simulink model "pibit_completo_2025_sem_obs_2025_2"  (R2025a)
settings: Solver=VariableStepAuto  StartTime=0.0  StopTime=10.0  RelTol=1e-3
values from neighbouring files (symbols this model uses):
  bp = 5    [parametros_suspensao_completo_pibit.m]    (also in parametros_suspensao_completo_pibit_final.m)
  bs = 10    [parametros_suspensao_completo_pibit.m]    (also in parametros_suspensao_completo_pibit_final.m)
  g = 9.81    [parametros_suspensao_completo_pibit.m]    (also in parametros_suspensao_completo_pibit_final.m)
  I = 5.6e-4    (= 0.00056)    [parametros_suspensao_completo_pibit.m]    (also in parametros_suspensao_completo_pibit_final.m)
  I_carroceria = (1/12) * m_carroceria * (L^2 + H^2)    (= 0.0082936384875)    [parametros_suspensao_completo_pibit_final.m]
  kp = 1000    [parametros_suspensao_completo_pibit.m]    (also in parametros_suspensao_completo_pibit_final.m)
  ks = 200    [parametros_suspensao_completo_pibit.m]    (also in parametros_suspensao_completo_pibit_final.m)
  M = [ ... (first row only)    [aprimorado_matlab_function_matriz_transformacao.m]    (also in bloco_matriz_tranformacao_pibit_final.m; bloco_matriz_tranformacao_pibit_semifinal.m; bloco_transposta_matriz_transformacao.m; matlab_function_matriz_transformacao.m)
  m_carroceria = 0.598725    [parametros_suspensao_completo_pibit_final.m]
  M_transposta = M'    [bloco_transposta_matriz_transformacao.m]    (also in parametros_suspensao_completo_pibit_final.m = [1  0  1  0  1)
  massa_nao_suspensa = 200/1000    (= 0.2)    [parametros_suspensao_completo_pibit.m]    (also in parametros_suspensao_completo_pibit_final.m)
  Vv = 5    [parametros_suspensao_completo_pibit_final.m]
  z0_carroceria = 0.12    [parametros_suspensao_completo_pibit_final.m]
  z0_roda = 0.04    [parametros_suspensao_completo_pibit_final.m]

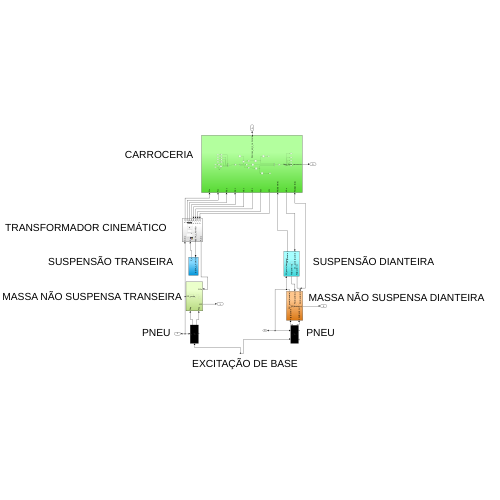
[thumbnail: Simulink's stored preview of the top-level diagram]
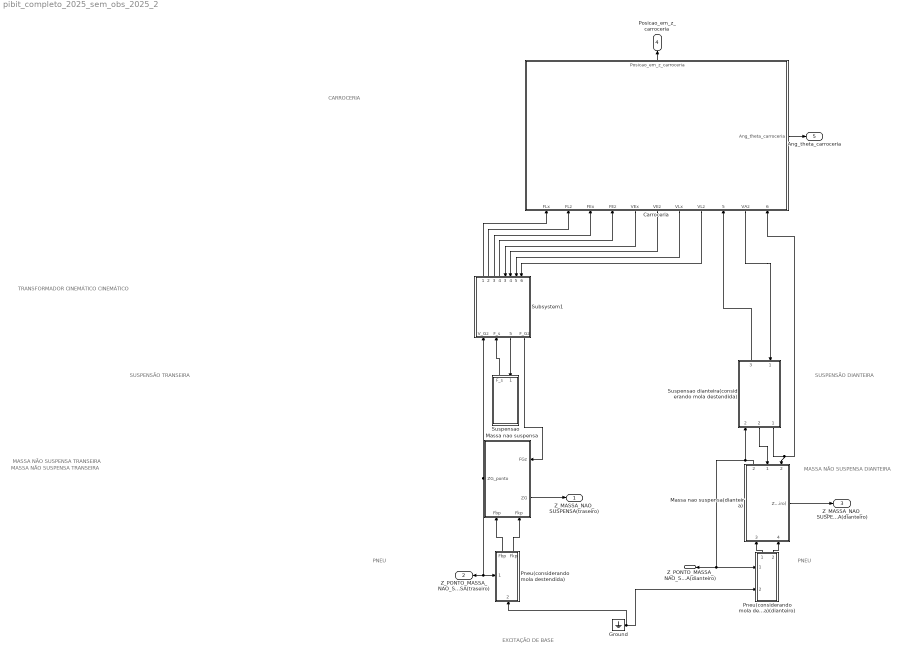
== system pibit_completo_2025_sem_obs_2025_2 ==
  note: MASSA NÃO SUSPENSA TRANSEIRA
  note: EXCITAÇÃO DE BASE
  note: SUSPENSÃO TRANSEIRA
  note: MASSA NÃO SUSPENSA DIANTEIRA
  note: SUSPENSÃO DIANTEIRA
  note: MASSA NÃO SUSPENSA TRANSEIRA
  note: CARROCERIA
  note: TRANSFORMADOR CINEMÁTICO
      |
      | CINEMÁTICO
  note: PNEU
  note: PNEU
  Carroceria : Subsystem
      settings: PortSchema="{\"entries\":[{\"content\":{\"sides\":[{\"content\":{},\"type\":\"ConnectorPlacement.EquallySpacedRectSide\",\"uuid\":\"bbb56681-fa3a-494c-b09e-961173c7fba7\"},{\"content\":{\"connectorIds\":[\"Out1\"],\"side\":\"RIGHT\"},\"type\":\"ConnectorPlacement.EquallySpacedRectSide\",\"uuid\":\"b39b7f7c-1399-4660-80c4-7db9c0d91b8e\"},{\"content\":{\"connectorIds\":[\"Out7\"],\"side\":\"TOP\"},\"type\":\"ConnectorPlacement.EquallySpacedRectSide\",\"uuid\":\"6aac35c2-b40a-442b-b0dd-a1f968c28842\"},{\"content\":{\"connectorIds\":[\"In1\",\"In2\",\"In3\",\"In4\",\"Out2\",\"Out3\",\"Out4\",\"Out5\",\"In5\",\"Out6\",\"In6\"],\"side\":\"BOTTOM\"},\"type\":\"ConnectorPlacement.EquallySpacedRectSide\",\"uuid\":\"4245813e-a678-4af8-87f3-459b1c319aee\"}]},\"type\":\"ConnectorPlacement.EquallySpacedConnector\",\"uuid\":\"f483dfe5-875a-4915-bcaf-a6efbf263f8a\"}],\"packageUris\":[\"http://schema.mathworks.com/mf0/Connector/R2020b\"],\"version\":\"1.0\"}"
  Ground : Ground
  Massa nao suspensa : Subsystem
      settings: PortSchema="{\"entries\":[{\"content\":{\"sides\":[{\"content\":{\"connectorIds\":[\"Out2\"]},\"type\":\"ConnectorPlacement.EquallySpacedRectSide\",\"uuid\":\"89344802-da43-4975-9b71-8316dc3fb6e7\"},{\"content\":{\"connectorIds\":[\"In3\",\"Out1\"],\"side\":\"RIGHT\"},\"type\":\"ConnectorPlacement.EquallySpacedRectSide\",\"uuid\":\"44d29e65-683b-44cb-8a4b-cd86ab3b5135\"},{\"content\":{\"side\":\"TOP\"},\"type\":\"ConnectorPlacement.EquallySpacedRectSide\",\"uuid\":\"980e030f-54fe-4b18-9c23-6eb2fde540e6\"},{\"content\":{\"connectorIds\":[\"In1\",\"In2\"],\"side\":\"BOTTOM\"},\"type\":\"ConnectorPlacement.EquallySpacedRectSide\",\"uuid\":\"baf76e64-0ac7-4a13-9c9f-461733e0ed7e\"}]},\"type\":\"ConnectorPlacement.EquallySpacedConnector\",\"uuid\":\"754d74c1-f226-49ce-a628-45964590b37b\"}],\"packageUris\":[\"http://schema.mathworks.com/mf0/Connector/R2020b\"],\"version\":\"1.0\"}"
  Massa nao suspensa(dianteira) : Subsystem
      settings: PortSchema="{\"entries\":[{\"content\":{\"sides\":[{\"content\":{},\"type\":\"ConnectorPlacement.EquallySpacedRectSide\",\"uuid\":\"c3cf290d-eebe-430e-95e8-be70dab148a6\"},{\"content\":{\"connectorIds\":[\"Out1\"],\"side\":\"RIGHT\"},\"type\":\"ConnectorPlacement.EquallySpacedRectSide\",\"uuid\":\"ff14580b-ed99-4b60-a1b6-b7a8b25b7868\"},{\"content\":{\"connectorIds\":[\"Out2\",\"In1\",\"In2\"],\"side\":\"TOP\"},\"type\":\"ConnectorPlacement.EquallySpacedRectSide\",\"uuid\":\"eb642ce5-fa56-48cf-87cc-3fd9675ce156\"},{\"content\":{\"connectorIds\":[\"In3\",\"In4\"],\"side\":\"BOTTOM\"},\"type\":\"ConnectorPlacement.EquallySpacedRectSide\",\"uuid\":\"0b9c6cb4-9fe7-4c64-813d-ec4cf3dc3e2a\"}]},\"type\":\"ConnectorPlacement.EquallySpacedConnector\",\"uuid\":\"a6d34252-cdb4-4e0a-800a-fcf48d8dc927\"}],\"packageUris\":[\"http://schema.mathworks.com/mf0/Connector/R2020b\"],\"version\":\"1.0\"}"
  Pneu(considerando mola destendida) : Subsystem
      settings: PortSchema="{\"entries\":[{\"content\":{\"sides\":[{\"content\":{\"connectorIds\":[\"In1\"]},\"type\":\"ConnectorPlacement.EquallySpacedRectSide\",\"uuid\":\"c5d69704-cabb-4fdd-98c1-bf4ac49d8bff\"},{\"content\":{\"side\":\"RIGHT\"},\"type\":\"ConnectorPlacement.EquallySpacedRectSide\",\"uuid\":\"557f2c7d-9be1-4292-a002-7cfc4acdfa17\"},{\"content\":{\"connectorIds\":[\"Out1\",\"Out2\"],\"side\":\"TOP\"},\"type\":\"ConnectorPlacement.EquallySpacedRectSide\",\"uuid\":\"4d76a2f1-24c8-44da-a892-d1fe66b59528\"},{\"content\":{\"connectorIds\":[\"In2\"],\"side\":\"BOTTOM\"},\"type\":\"ConnectorPlacement.EquallySpacedRectSide\",\"uuid\":\"89b6f56a-af2b-419d-a0b0-9e96ef479f92\"}]},\"type\":\"ConnectorPlacement.EquallySpacedConnector\",\"uuid\":\"f14e1ba1-d9bd-4a41-a66d-11d76b469bcb\"}],\"packageUris\":[\"http://schema.mathworks.com/mf0/Connector/R2020b\"],\"version\":\"1.0\"}"
  Pneu(considerando mola destendida)(dianteiro) : Subsystem
      settings: PortSchema="{\"entries\":[{\"content\":{\"sides\":[{\"content\":{\"connectorIds\":[\"In1\",\"In2\"]},\"type\":\"ConnectorPlacement.EquallySpacedRectSide\",\"uuid\":\"c5d69704-cabb-4fdd-98c1-bf4ac49d8bff\"},{\"content\":{\"side\":\"RIGHT\"},\"type\":\"ConnectorPlacement.EquallySpacedRectSide\",\"uuid\":\"557f2c7d-9be1-4292-a002-7cfc4acdfa17\"},{\"content\":{\"connectorIds\":[\"Out1\",\"Out2\"],\"side\":\"TOP\"},\"type\":\"ConnectorPlacement.EquallySpacedRectSide\",\"uuid\":\"4d76a2f1-24c8-44da-a892-d1fe66b59528\"}]},\"type\":\"ConnectorPlacement.EquallySpacedConnector\",\"uuid\":\"f14e1ba1-d9bd-4a41-a66d-11d76b469bcb\"}],\"packageUris\":[\"http://schema.mathworks.com/mf0/Connector/R2020b\"],\"version\":\"1.0\"}"
  Subsystem1 : Subsystem
      settings: PortSchema="{\"entries\":[{\"content\":{\"sides\":[{\"content\":{\"connectorIds\":[\"In1\",\"In2\",\"Out5\",\"Out6\"]},\"type\":\"ConnectorPlacement.EquallySpacedRectSide\",\"uuid\":\"bebb3b97-f51a-4e56-a2ac-0bf355c169a6\"},{\"content\":{\"connectorIds\":[\"Out1\",\"Out2\",\"Out3\",\"Out4\",\"In3\",\"In4\",\"In5\",\"In6\"],\"side\":\"RIGHT\"},\"type\":\"ConnectorPlacement.EquallySpacedRectSide\",\"uuid\":\"70a45981-1049-4317-936c-533ae84876c2\"},{\"content\":{\"side\":\"TOP\"},\"type\":\"ConnectorPlacement.EquallySpacedRectSide\",\"uuid\":\"f9228920-a333-4bb0-97b2-e9b2d0e5e8fb\"}]},\"type\":\"ConnectorPlacement.EquallySpacedConnector\",\"uuid\":\"080e89e8-39a4-4dac-ac05-f09c1a8f52a2\"}],\"packageUris\":[\"http://schema.mathworks.com/mf0/Connector/R2020b\"],\"version\":\"1.0\"}"
  Suspensao : Subsystem
      settings: PortSchema="{\"entries\":[{\"content\":{\"sides\":[{\"content\":{},\"type\":\"ConnectorPlacement.EquallySpacedRectSide\",\"uuid\":\"4f1921ee-033d-46ee-8e73-30eca5c2181d\"},{\"content\":{\"side\":\"RIGHT\"},\"type\":\"ConnectorPlacement.EquallySpacedRectSide\",\"uuid\":\"dda2b99d-9329-4e8f-bdf2-d73cce971ac2\"},{\"content\":{\"connectorIds\":[\"In1\",\"Out1\"],\"side\":\"TOP\"},\"type\":\"ConnectorPlacement.EquallySpacedRectSide\",\"uuid\":\"e9d42515-3d20-42dd-b281-3c9bfd9b1cfa\"},{\"content\":{\"side\":\"BOTTOM\"},\"type\":\"ConnectorPlacement.EquallySpacedRectSide\",\"uuid\":\"bd1a0df3-c979-436b-84b6-72c0af110375\"}]},\"type\":\"ConnectorPlacement.EquallySpacedConnector\",\"uuid\":\"cbab4240-af80-4068-bc0e-573c06bf1f73\"}],\"packageUris\":[\"http://schema.mathworks.com/mf0/Connector/R2020b\"],\"version\":\"1.0\"}"
  Suspensao dianteira(considerando mola destendida) : Subsystem
      settings: PortSchema="{\"entries\":[{\"content\":{\"sides\":[{\"content\":{\"connectorIds\":[\"In1\",\"Out3\"]},\"type\":\"ConnectorPlacement.EquallySpacedRectSide\",\"uuid\":\"d327c13d-9315-480e-be5c-199a2935ffa2\"},{\"content\":{\"connectorIds\":[\"Out1\",\"Out2\",\"In2\"],\"side\":\"RIGHT\"},\"type\":\"ConnectorPlacement.EquallySpacedRectSide\",\"uuid\":\"b456819d-8f70-476a-8897-c81e34c4473c\"},{\"content\":{\"side\":\"TOP\"},\"type\":\"ConnectorPlacement.EquallySpacedRectSide\",\"uuid\":\"b01201ff-aebb-430e-af55-356b9f96849b\"}]},\"type\":\"ConnectorPlacement.EquallySpacedConnector\",\"uuid\":\"690aae98-0b40-4873-810d-deff39bc59c7\"}],\"packageUris\":[\"http://schema.mathworks.com/mf0/Connector/R2020b\"],\"version\":\"1.0\"}"
  Z_MASSA_NAO_SUSPENSA(traseiro) : Outport
  Z_PONTO_MASSA_NAO_SUSPENSA(traseiro) : Outport  Port=2
  Z_MASSA_NAO_SUSPENSA(dianteiro) : Outport  Port=3
  Posicao_em_z_carroceria : Outport  Port=4
  Ang_theta_carroceria : Outport  Port=5
  Z_PONTO_MASSA_NAO_SUSPENSA(dianteiro) : Outport  Port=6
  wires:
  Subsystem1/1(F_Lx) -> Carroceria/1(FLx)
  Massa nao suspensa/1(ZG) -> Z_MASSA_NAO_SUSPENSA(traseiro)/1
  Pneu(considerando mola destendida)(dianteiro)/2(Fbp(dianteiro)) -> Massa nao suspensa(dianteira)/4(Fbp(dianteiro))
  Massa nao suspensa/2(ZG_ponto) -> Z_PONTO_MASSA_NAO_SUSPENSA(traseiro)/1, Pneu(considerando mola destendida)/1(ZG_ponto), Subsystem1/1(V_Gz)
  Suspensao dianteira(considerando mola destendida)/2(Fk(dianteiro)1) -> Massa nao suspensa(dianteira)/1(Fb(dianteiro)1)
  Suspensao/1(F_s) -> Subsystem1/2(F_s)
  Massa nao suspensa(dianteira)/2(ZG_ponto(dianteiro)) -> Suspensao dianteira(considerando mola destendida)/2(ZG_ponto(dianteiro)), Z_PONTO_MASSA_NAO_SUSPENSA(dianteiro)/1, Pneu(considerando mola destendida)(dianteiro)/1(ZG_ponto(dianteiro))
  Suspensao dianteira(considerando mola destendida)/3(Fb(dianteiro)) -> Carroceria/5(Fb(dianteiro))
  Subsystem1/6(F_Gz) -> Massa nao suspensa/3(FGz)
  Subsystem1/4(F_Ez) -> Carroceria/4(FEz)
  Subsystem1/3(F_Ex) -> Carroceria/3(FEx)
  Carroceria/1(Ang_theta_carroceria) -> Ang_theta_carroceria/1
  Carroceria/6(VAz) -> Suspensao dianteira(considerando mola destendida)/1(ZA_ponto(dianteiro))
  Carroceria/7(Posicao_em_z_carroceria) -> Posicao_em_z_carroceria/1
  Carroceria/2(VEx) -> Subsystem1/3(V_Ex)
  Pneu(considerando mola destendida)(dianteiro)/1(Fkp(dianteiro)) -> Massa nao suspensa(dianteira)/3(Fkp(dianteiro))
  Carroceria/5(VLz) -> Subsystem1/6(V_Lz)
  Carroceria/4(VLx) -> Subsystem1/5(V_Lx)
  Suspensao dianteira(considerando mola destendida)/1(Fk(dianteiro)) -> Massa nao suspensa(dianteira)/2(Fk(dianteiro)2), Carroceria/6(Fk(dianteiro))
  Carroceria/3(VEz) -> Subsystem1/4(V_Ez)
  Subsystem1/5(BETA_1_PONTO) -> Suspensao/1(BETA_1_PONTO)
  Massa nao suspensa(dianteira)/1(ZG(dianteiro)) -> Z_MASSA_NAO_SUSPENSA(dianteiro)/1
  Pneu(considerando mola destendida)/2(Fkp) -> Massa nao suspensa/2(Fkp)
  Subsystem1/2(F_Lz) -> Carroceria/2(FLz)
  Pneu(considerando mola destendida)/1(Fbp) -> Massa nao suspensa/1(Fbp)
  Ground/1 -> Pneu(considerando mola destendida)/2(Z1_ponto), Pneu(considerando mola destendida)(dianteiro)/2(Z1_ponto(dianteiro))

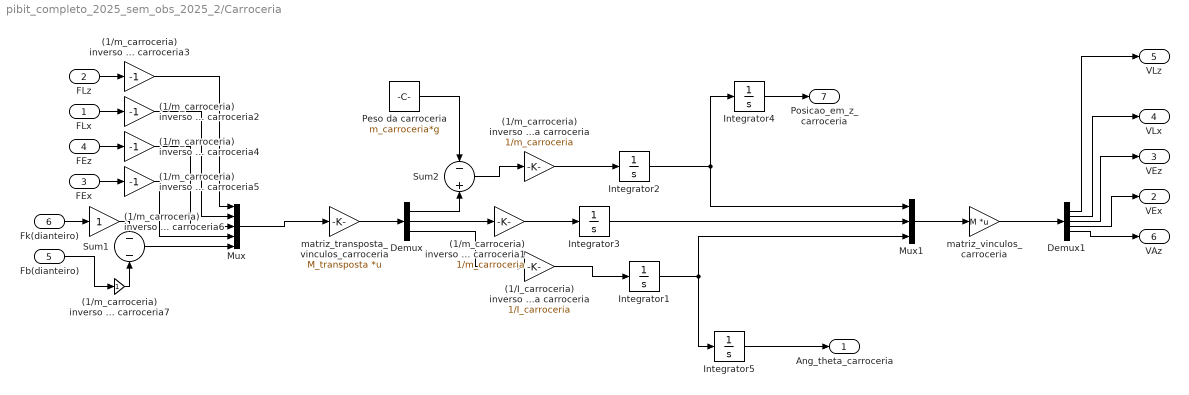
== system pibit_completo_2025_sem_obs_2025_2/Carroceria ==
  FLx : Inport
  FLz : Inport  Port=2
  FEx : Inport  Port=3
  FEz : Inport  Port=4
  Fb(dianteiro) : Inport  Port=5
  Fk(dianteiro) : Inport  Port=6
  (1/I_carroceria) inverso do momento de inercia da carroceria : Gain  Gain=1/I_carroceria
  (1/m_carroceria) inverso da massa da carroceria : Gain  Gain=1/m_carroceria
  (1/m_carroceria) inverso da massa da carroceria1 : Gain  Gain=1/m_carroceria
  (1/m_carroceria) inverso da massa da carroceria{2..5} (4 alike) : Gain  Gain=-1
  (1/m_carroceria) inverso da massa da carroceria6 : Gain
  (1/m_carroceria) inverso da massa da carroceria7 : Gain
  Demux : Demux  Outputs=3
  Demux1 : Demux  Outputs=5
  Integrator1 : Integrator
  Integrator2 : Integrator
  Integrator3 : Integrator  InitialCondition=Vv
  Integrator4 : Integrator  InitialCondition=z0_carroceria
  Integrator5 : Integrator
  Mux : Mux  Inputs=5
  Mux1 : Mux  Inputs=3
  Peso da carroceria : Constant  Value=m_carroceria*g
  Sum1 : Sum  Inputs=--
  Sum2 : Sum  Inputs=-+
  matriz_transposta_vinculos_carroceria : Gain  Gain=M_transposta  Multiplication=Matrix(K*u) (u vector)
  matriz_vinculos_carroceria : Gain  Gain=M  Multiplication=Matrix(K*u) (u vector)
  Ang_theta_carroceria : Outport
  VEx : Outport  Port=2
  VEz : Outport  Port=3
  VLx : Outport  Port=4
  VLz : Outport  Port=5
  VAz : Outport  Port=6
  Posicao_em_z_carroceria : Outport  Port=7
  wires:
  Fk(dianteiro)/1 -> (1/m_carroceria) inverso da massa da carroceria6/1
  Fb(dianteiro)/1 -> (1/m_carroceria) inverso da massa da carroceria7/1
  FLz/1 -> (1/m_carroceria) inverso da massa da carroceria3/1
  FLx/1 -> (1/m_carroceria) inverso da massa da carroceria2/1
  FEz/1 -> (1/m_carroceria) inverso da massa da carroceria4/1
  FEx/1 -> (1/m_carroceria) inverso da massa da carroceria5/1
  Sum1/1 -> Mux/5
  Mux/1 -> matriz_transposta_vinculos_carroceria/1
  matriz_transposta_vinculos_carroceria/1 -> Demux/1
  Peso da carroceria/1 -> Sum2/1
  Demux/1 -> Sum2/2
  Sum2/1 -> (1/m_carroceria) inverso da massa da carroceria/1
  (1/m_carroceria) inverso da massa da carroceria/1 -> Integrator2/1
  Demux/2 -> (1/m_carroceria) inverso da massa da carroceria1/1
  Demux/3 -> (1/I_carroceria) inverso do momento de inercia da carroceria/1
  (1/I_carroceria) inverso do momento de inercia da carroceria/1 -> Integrator1/1
  (1/m_carroceria) inverso da massa da carroceria1/1 -> Integrator3/1
  Integrator2/1 -> Integrator4/1, Mux1/1
  Mux1/1 -> matriz_vinculos_carroceria/1
  matriz_vinculos_carroceria/1 -> Demux1/1
  Demux1/1 -> VLz/1
  Demux1/2 -> VLx/1
  Demux1/3 -> VEz/1
  Demux1/4 -> VEx/1
  Demux1/5 -> VAz/1
  Integrator1/1 -> Integrator5/1, Mux1/3
  (1/m_carroceria) inverso da massa da carroceria3/1 -> Mux/1
  (1/m_carroceria) inverso da massa da carroceria2/1 -> Mux/2
  (1/m_carroceria) inverso da massa da carroceria4/1 -> Mux/3
  (1/m_carroceria) inverso da massa da carroceria5/1 -> Mux/4
  (1/m_carroceria) inverso da massa da carroceria6/1 -> Sum1/1
  (1/m_carroceria) inverso da massa da carroceria7/1 -> Sum1/2
  Integrator3/1 -> Mux1/2
  Integrator4/1 -> Posicao_em_z_carroceria/1
  Integrator5/1 -> Ang_theta_carroceria/1

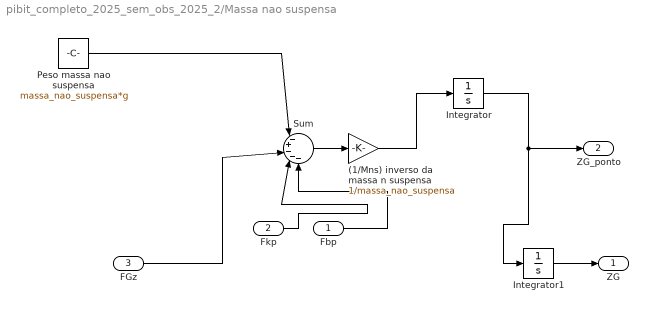
== system pibit_completo_2025_sem_obs_2025_2/Massa nao suspensa ==
  Fbp : Inport
  Fkp : Inport  Port=2
  FGz : Inport  Port=3
  (1/Mns) inverso da massa n suspensa : Gain  Gain=1/massa_nao_suspensa
  Integrator : Integrator
  Integrator1 : Integrator  InitialCondition=z0_roda
  Peso massa nao suspensa : Constant  Value=massa_nao_suspensa*g
  Sum : Sum  Inputs=|-+---
  ZG : Outport
  ZG_ponto : Outport  Port=2
  wires:
  Integrator/1 -> Integrator1/1, ZG_ponto/1
  Fbp/1 -> Sum/5
  Fkp/1 -> Sum/4
  (1/Mns) inverso da massa n suspensa/1 -> Integrator/1
  Sum/1 -> (1/Mns) inverso da massa n suspensa/1
  FGz/1 -> Sum/3
  Integrator1/1 -> ZG/1
  Peso massa nao suspensa/1 -> Sum/1

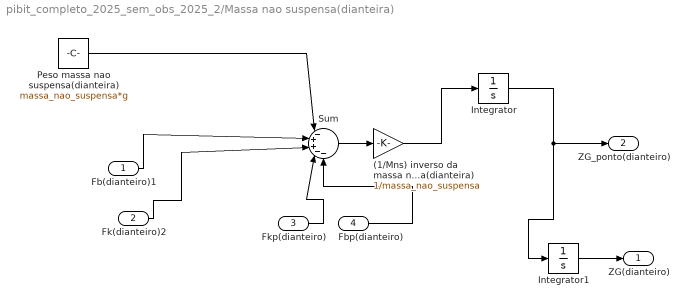
== system pibit_completo_2025_sem_obs_2025_2/Massa nao suspensa(dianteira) ==
  Fb(dianteiro)1 : Inport
  Fk(dianteiro)2 : Inport  Port=2
  Fkp(dianteiro) : Inport  Port=3
  Fbp(dianteiro) : Inport  Port=4
  (1/Mns) inverso da massa nao suspensa(dianteira) : Gain  Gain=1/massa_nao_suspensa
  Integrator : Integrator
  Integrator1 : Integrator  InitialCondition=z0_roda
  Peso massa nao suspensa(dianteira) : Constant  Value=massa_nao_suspensa*g
  Sum : Sum  Inputs=|-++--
  ZG(dianteiro) : Outport
  ZG_ponto(dianteiro) : Outport  Port=2
  wires:
  Integrator/1 -> Integrator1/1, ZG_ponto(dianteiro)/1
  Fbp(dianteiro)/1 -> Sum/5
  Fkp(dianteiro)/1 -> Sum/4
  (1/Mns) inverso da massa nao suspensa(dianteira)/1 -> Integrator/1
  Sum/1 -> (1/Mns) inverso da massa nao suspensa(dianteira)/1
  Integrator1/1 -> ZG(dianteiro)/1
  Fb(dianteiro)1/1 -> Sum/2
  Fk(dianteiro)2/1 -> Sum/3
  Peso massa nao suspensa(dianteira)/1 -> Sum/1

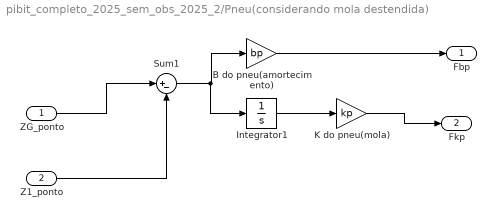
== system pibit_completo_2025_sem_obs_2025_2/Pneu(considerando mola destendida) ==
  ZG_ponto : Inport
  Z1_ponto : Inport  Port=2
  B do pneu(amortecimento) : Gain  Gain=bp
  Integrator1 : Integrator
  K do pneu(mola) : Gain  Gain=kp
  Sum1 : Sum  Inputs=|+-
  Fbp : Outport
  Fkp : Outport  Port=2
  wires:
  Z1_ponto/1 -> Sum1/2
  ZG_ponto/1 -> Sum1/1
  Sum1/1 -> Integrator1/1, B do pneu(amortecimento)/1
  K do pneu(mola)/1 -> Fkp/1
  B do pneu(amortecimento)/1 -> Fbp/1
  Integrator1/1 -> K do pneu(mola)/1

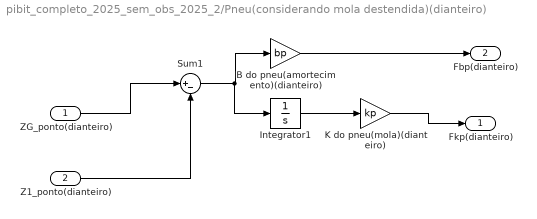
== system pibit_completo_2025_sem_obs_2025_2/Pneu(considerando mola destendida)(dianteiro) ==
  ZG_ponto(dianteiro) : Inport
  Z1_ponto(dianteiro) : Inport  Port=2
  B do pneu(amortecimento)(dianteiro) : Gain  Gain=bp
  Integrator1 : Integrator
  K do pneu(mola)(dianteiro) : Gain  Gain=kp
  Sum1 : Sum  Inputs=|+-
  Fkp(dianteiro) : Outport
  Fbp(dianteiro) : Outport  Port=2
  wires:
  Z1_ponto(dianteiro)/1 -> Sum1/2
  ZG_ponto(dianteiro)/1 -> Sum1/1
  Sum1/1 -> Integrator1/1, B do pneu(amortecimento)(dianteiro)/1
  K do pneu(mola)(dianteiro)/1 -> Fkp(dianteiro)/1
  B do pneu(amortecimento)(dianteiro)/1 -> Fbp(dianteiro)/1
  Integrator1/1 -> K do pneu(mola)(dianteiro)/1

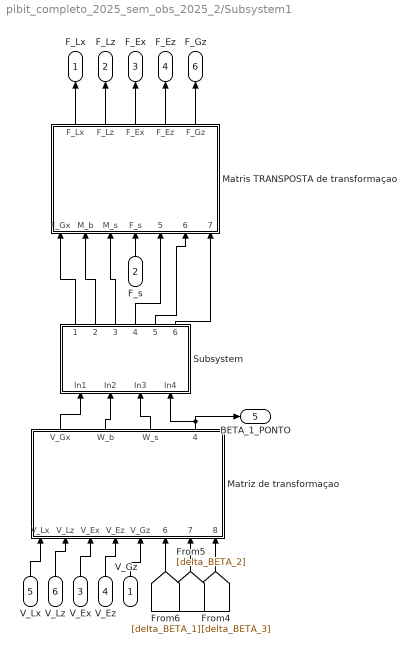
== system pibit_completo_2025_sem_obs_2025_2/Subsystem1 ==
  V_Gz : Inport
  F_s : Inport  Port=2
  V_Ex : Inport  Port=3
  V_Ez : Inport  Port=4
  V_Lx : Inport  Port=5
  V_Lz : Inport  Port=6
  Matris TRANSPOSTA de transformaçao : MATLAB Function  TreatAsAtomicUnit=on
  Matriz de transformaçao : MATLAB Function  TreatAsAtomicUnit=on
  Subsystem : Subsystem
  F_Lx : Outport
  F_Lz : Outport  Port=2
  F_Ex : Outport  Port=3
  F_Ez : Outport  Port=4
  BETA_1_PONTO : Outport  Port=5
  F_Gz : Outport  Port=6
  wires:
  V_Ex/1 -> Matriz de transformaçao/3(V_Ex)
  [delta_BETA_2] -> Matriz de transformaçao/7(delta_BETA_2)
  Subsystem/1(Out1) -> Matris TRANSPOSTA de transformaçao/1(F_Gx)
  [delta_BETA_1] -> Matriz de transformaçao/6(delta_BETA_1)
  [delta_BETA_3] -> Matriz de transformaçao/8(delta_BETA_3)
  Subsystem/2(Out2) -> Matris TRANSPOSTA de transformaçao/2(M_b)
  Matriz de transformaçao/2(W_b) -> Subsystem/2(In2)
  V_Lz/1 -> Matriz de transformaçao/2(V_Lz)
  Matris TRANSPOSTA de transformaçao/5(F_Gz) -> F_Gz/1
  Matriz de transformaçao/1(V_Gx) -> Subsystem/1(In1)
  Subsystem/4(Out4) -> Matris TRANSPOSTA de transformaçao/5(delta_BETA_1)
  V_Gz/1 -> Matriz de transformaçao/5(V_Gz)
  Matris TRANSPOSTA de transformaçao/1(F_Lx) -> F_Lx/1
  Matris TRANSPOSTA de transformaçao/2(F_Lz) -> F_Lz/1
  V_Lx/1 -> Matriz de transformaçao/1(V_Lx)
  F_s/1 -> Matris TRANSPOSTA de transformaçao/4(F_s)
  Subsystem/3(Out3) -> Matris TRANSPOSTA de transformaçao/3(M_s)
  Matriz de transformaçao/4(BETA_1_PONTO) -> BETA_1_PONTO/1, Subsystem/4(In4)
  Subsystem/5(Out5) -> Matris TRANSPOSTA de transformaçao/6(delta_BETA_2)
  Matris TRANSPOSTA de transformaçao/3(F_Ex) -> F_Ex/1
  Matriz de transformaçao/3(W_s) -> Subsystem/3(In3)
  Matris TRANSPOSTA de transformaçao/4(F_Ez) -> F_Ez/1
  V_Ez/1 -> Matriz de transformaçao/4(V_Ez)
  Subsystem/6(Out6) -> Matris TRANSPOSTA de transformaçao/7(delta_BETA_3)

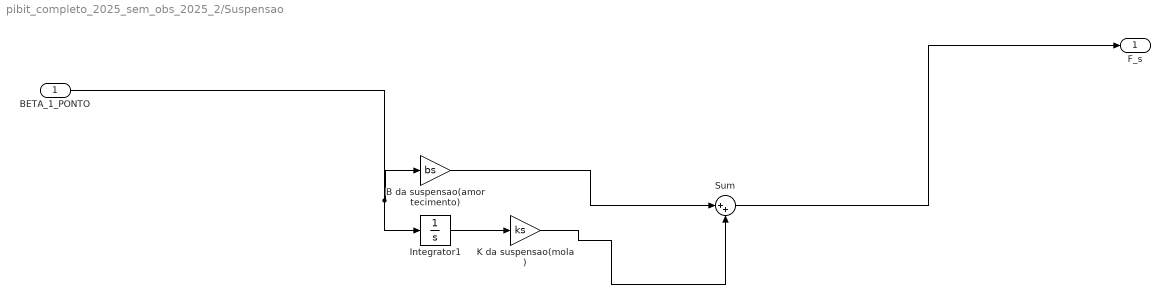
== system pibit_completo_2025_sem_obs_2025_2/Suspensao ==
  BETA_1_PONTO : Inport
  B da suspensao(amortecimento) : Gain  Gain=bs
  Integrator1 : Integrator
  K da suspensao(mola) : Gain  Gain=ks
  Sum : Sum  Inputs=|++
  F_s : Outport
  wires:
  K da suspensao(mola)/1 -> Sum/2
  Sum/1 -> F_s/1
  B da suspensao(amortecimento)/1 -> Sum/1
  Integrator1/1 -> K da suspensao(mola)/1
  BETA_1_PONTO/1 -> Integrator1/1, B da suspensao(amortecimento)/1

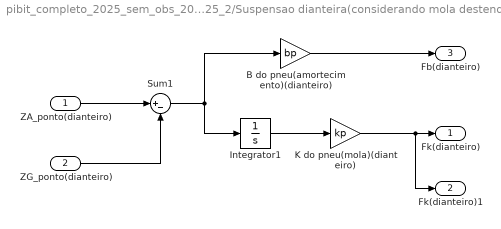
== system pibit_completo_2025_sem_obs_2025_2/Suspensao dianteira(considerando mola destendida) ==
  ZA_ponto(dianteiro) : Inport
  ZG_ponto(dianteiro) : Inport  Port=2
  B do pneu(amortecimento)(dianteiro) : Gain  Gain=bp
  Integrator1 : Integrator
  K do pneu(mola)(dianteiro) : Gain  Gain=kp
  Sum1 : Sum  Inputs=|+-
  Fk(dianteiro) : Outport
  Fk(dianteiro)1 : Outport  Port=2
  Fb(dianteiro) : Outport  Port=3
  wires:
  ZG_ponto(dianteiro)/1 -> Sum1/2
  ZA_ponto(dianteiro)/1 -> Sum1/1
  Sum1/1 -> Integrator1/1, B do pneu(amortecimento)(dianteiro)/1
  K do pneu(mola)(dianteiro)/1 -> Fk(dianteiro)1/1, Fk(dianteiro)/1
  B do pneu(amortecimento)(dianteiro)/1 -> Fb(dianteiro)/1
  Integrator1/1 -> K do pneu(mola)(dianteiro)/1

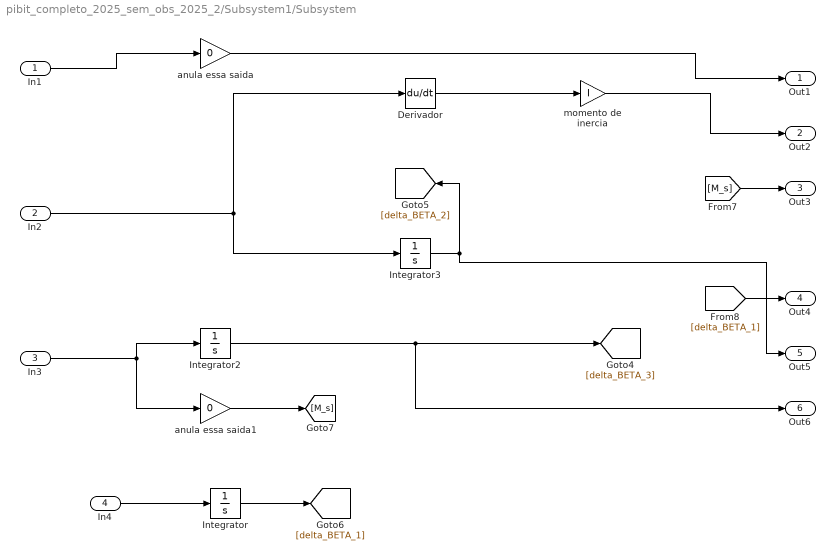
== system pibit_completo_2025_sem_obs_2025_2/Subsystem1/Subsystem ==
  In1 : Inport
  In2 : Inport  Port=2
  In3 : Inport  Port=3
  In4 : Inport  Port=4
  Derivador : Derivative
  Integrator : Integrator
  Integrator2 : Integrator
  Integrator3 : Integrator
  anula essa saida : Gain  Gain=0
  anula essa saida1 : Gain  Gain=0
  momento de inercia : Gain  Gain=I
  Out1 : Outport
  Out2 : Outport  Port=2
  Out3 : Outport  Port=3
  Out4 : Outport  Port=4
  Out5 : Outport  Port=5
  Out6 : Outport  Port=6
  wires:
  Integrator/1 -> [delta_BETA_1]
  Integrator2/1 -> Out6/1, [delta_BETA_3]
  In1/1 -> anula essa saida/1
  In4/1 -> Integrator/1
  Derivador/1 -> momento de inercia/1
  [M_s] -> Out3/1
  anula essa saida1/1 -> [M_s]
  anula essa saida/1 -> Out1/1
  In2/1 -> Derivador/1, Integrator3/1
  In3/1 -> Integrator2/1, anula essa saida1/1
  momento de inercia/1 -> Out2/1
  Integrator3/1 -> Out5/1, [delta_BETA_2]
  [delta_BETA_1] -> Out4/1

== matlab function pibit_completo_2025_sem_obs_2025_2/Subsystem1/Matris TRANSPOSTA de transformaçao ==
  data: F_Gx input; F_Lx output; M_b input; M_s input; F_s input; F_Lz output; F_Ex output; F_Ez output; F_Gz output; delta_BETA_1 input; delta_BETA_2 input; delta_BETA_3 input

function [F_Lx, F_Lz, F_Ex, F_Ez, F_Gz] = minhaFuncaoForcas( ...
    F_Gx, M_b, M_s, F_s, delta_BETA_1, delta_BETA_2, delta_BETA_3)

    % Valores nominais iniciais
    BETA_1_0 = 0.055;
    BETA_2_0 = 2.6;
    BETA_3_0 = 2.2;

    % Limites físicos dos parâmetros
    BETA_1_min = 0.05465;
    BETA_1_max = 0.0589;
    BETA_2_min = 2.591;
    BETA_2_max = 2.729;
    BETA_3_min = 2.168;
    BETA_3_max = 2.264;

    % Atualização com limite (clamping)
    BETA_1 = min(max(BETA_1_0 + delta_BETA_1, BETA_1_min), BETA_1_max);
    BETA_2 = min(max(BETA_2_0 + delta_BETA_2, BETA_2_min), BETA_2_max);
    BETA_3 = min(max(BETA_3_0 + delta_BETA_3, BETA_3_min), BETA_3_max);

    % Constantes fixas
    GAMA = 0.380;
    R_1 = 0.091782;
    R_2 = 0.048414;

    % Matriz M atualizada
    M = [
        0, 0, 1, -tan(BETA_2), tan(BETA_2);
        0, 0, 0, 1 / (R_1 * cos(BETA_2)), -1 / (R_1 * cos(BETA_2));
        sin(BETA_3) / BETA_1, cos(BETA_3) / BETA_1, -sin(BETA_3) / BETA_1, ...
        (R_2 * cos(BETA_2 + GAMA - BETA_3) / (R_1 * cos(BETA_2) * BETA_1)) - cos(BETA_3) / BETA_1, ...
        -R_2 * cos(BETA_2 + GAMA - BETA_3) / (R_1 * cos(BETA_2) * BETA_1);
        -cos(BETA_3), sin(BETA_3), cos(BETA_3), ...
        (R_2 * sin(-(BETA_2 + GAMA) + BETA_3) / (R_1 * cos(BETA_2))) - sin(BETA_3), ...
        R_2 * sin((BETA_2 + GAMA) - BETA_3) / (R_1 * cos(BETA_2))
    ];

    % Matriz transposta
    M_transposta = M';

    % Cálculo do resultado
    resultado = M_transposta * [F_Gx; M_b; M_s; F_s];

    % Saídas
    F_Lx = resultado(1);
    F_Lz = resultado(2);
    F_Ex = resultado(3);
    F_Ez = resultado(4);
    F_Gz = resultado(5);
end

== matlab function pibit_completo_2025_sem_obs_2025_2/Subsystem1/Matriz de transformaçao ==
  data: V_Lx input; V_Gx output; V_Lz input; V_Ex input; V_Ez input; V_Gz input; W_b output; W_s output; BETA_1_PONTO output; delta_BETA_1 input; delta_BETA_2 input; delta_BETA_3 input
function [V_Gx, W_b, W_s, BETA_1_PONTO] = fcn( ...
    V_Lx, V_Lz, V_Ex, V_Ez, V_Gz, ...
    delta_BETA_1, delta_BETA_2, delta_BETA_3)

% Valores nominais (iniciais)
BETA_1_0 = 0.055;
BETA_2_0 = 2.6;
BETA_3_0 = 2.2;

% Limites físicos dos parâmetros
BETA_1_min = 0.05465;
BETA_1_max = 0.0589;
BETA_2_min = 2.591;
BETA_2_max = 2.729;
BETA_3_min = 2.168;
BETA_3_max = 2.264;

% Atualização dos parâmetros
BETA_1 = min(max(BETA_1_0 + delta_BETA_1, BETA_1_min), BETA_1_max);
BETA_2 = min(max(BETA_2_0 + delta_BETA_2, BETA_2_min), BETA_2_max);
BETA_3 = min(max(BETA_3_0 + delta_BETA_3, BETA_3_min), BETA_3_max);

% Constantes
GAMA = 0.380;
R_1 = 0.091782;
R_2 = 0.048414;

% Matriz M
M = [
    0, 0, 1, -tan(BETA_2), tan(BETA_2);
    0, 0, 0, 1 / (R_1 * cos(BETA_2)), -1 / (R_1 * cos(BETA_2));
    sin(BETA_3) / BETA_1, cos(BETA_3) / BETA_1, -sin(BETA_3) / BETA_1, ...
    (R_2 * cos(BETA_2 + GAMA - BETA_3) / (R_1 * cos(BETA_2) * BETA_1)) - cos(BETA_3) / BETA_1, ...
    -R_2 * cos(BETA_2 + GAMA - BETA_3) / (R_1 * cos(BETA_2) * BETA_1);
    -cos(BETA_3), sin(BETA_3), cos(BETA_3), ...
    (R_2 * sin(-(BETA_2 + GAMA) + BETA_3) / (R_1 * cos(BETA_2))) - sin(BETA_3), ...
    R_2 * sin((BETA_2 + GAMA) - BETA_3) / (R_1 * cos(BETA_2))
];

entrada = [V_Lx; V_Lz; V_Ex; V_Ez; V_Gz];
resultado = M * entrada;

% Saídas
V_Gx         = resultado(1);
W_b          = resultado(2);
W_s          = resultado(3);
BETA_1_PONTO = resultado(4);
